simulink model "UWSim_test"  (R2018b)
settings: Solver=VariableStepAuto  StartTime=0.0  StopTime=10.0  RelTol=1e-3
libraries: simulink x6, robotlib x4
settings Model: Creator=carter  LastModifiedBy=carter

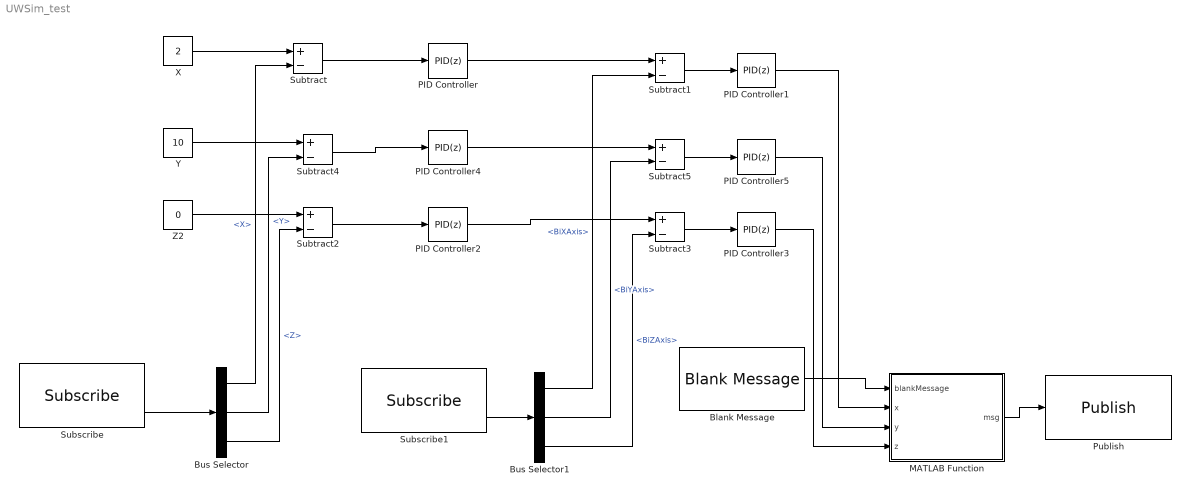
== system UWSim_test ==
  Blank Message : robotlib/Blank Message  messageClass=Message  entityType=std_msgs/Float64MultiArray  messageType=std_msgs/Float64MultiArray  SampleTime=1/50
      settings: SourceProductBaseCode=RO
  Bus Selector : BusSelector  OutputSignals=Position.X,Position.Y,Position.Z
  Bus Selector1 : BusSelector  OutputSignals=BiXAxis,BiYAxis,BiZAxis
  MATLAB Function : MATLAB Function  TreatAsAtomicUnit=on
  PID Controller{,1..5} (6 alike) : simulink/Continuous/PID Controller  Controller=PID  Form=Parallel  TimeDomain=Discrete-time  SampleTime=1/50  IntegratorMethod=Forward Euler  FilterMethod=Forward Euler  ControllerParametersSource=internal  P=0.5  I=0  D=0  UseFilter=on  N=100  TunerSelectOption=Transfer Function Based (PID Tuner App)  InitialConditionSource=internal  InitialConditionForIntegrator=0  InitialConditionForFilter=0  DifferentiatorICPrevScaledInput=0  ExternalReset=none  TrackingMode=off  Kt=1  LimitOutput=off  UpperSaturationLimit=inf  LowerSaturationLimit=-inf  LinearizeAsGain=on  AntiWindupMode=none  Kb=1  POutMin=[]  POutMax=[]  IOutMin=[]  IOutMax=[]  DOutMin=[]  DOutMax=[]  NOutMin=[]  NOutMax=[]  SumOutMin=[]  SumOutMax=[]  SaturationOutMin=[]  SaturationOutMax=[]  PParamMin=[]  PParamMax=[]  IParamMin=[]  IParamMax=[]  DParamMin=[]  DParamMax=[]  NParamMin=[]  NParamMax=[]  KbParamMin=[]  KbParamMax=[]  KtParamMin=[]  KtParamMax=[]  KbOutMin=[]  KbOutMax=[]  KtOutMin=[]  KtOutMax=[]  IntegratorOutMin=[]  IntegratorOutMax=[]  FilterOutMin=[]  FilterOutMax=[]  SumI1OutMin=[]  SumI1OutMax=[]  SumI2OutMin=[]  SumI2OutMax=[]  SumI3OutMin=[]  SumI3OutMax=[]  SumI4OutMin=[]  SumI4OutMax=[]  SumDOutMin=[]  SumDOutMax=[]  DifferentiatorOutMin=[]  DifferentiatorOutMax=[]  FilterDiffOutCoefMin=[]  FilterDiffOutCoefMax=[]  ReciprocalOutMin=[]  ReciprocalOutMax=[]  SumDenOutMin=[]  SumDenOutMax=[]  SumNumOutMin=[]  SumNumOutMax=[]  DivideOutMin=[]  DivideOutMax=[]  IntegratorContinuousStateAttributes=''  IntegratorStateMustResolveToSignalObject=off  IntegratorRTWStateStorageClass=Auto  FilterContinuousStateAttributes=''  FilterStateMustResolveToSignalObject=off  FilterRTWStateStorageClass=Auto  ParallelPVariant=InternalParameters  IdealPVariant=Disabled  IVariant=InternalParameters  DVariant=InternalParameters  IntegratorVariant=Discrete  SatVariant=Disabled  AWVariant=Passthrough  PCopyVariant=Disabled  TRVariant=Disabled  FdbkBlocksVariant=Forward  IdealPFdbkVariant=Disabled  SatFdbkVariant=Disabled  DerivativeFilterVariant=ForwardEulerFilter  NVariant=InternalParameters  NCopyVariant=Disabled  FilterICVariant=InternalICsFilter  IntegratorICVariant=InternalICs  ExternalResetVariant=Disabled  TRSumVariant=Passthrough  SumFdbkVariant=Disabled  SumVariant=Sum_PID
  Publish : robotlib/Publish  topicSource=Select from ROS network  topic=/g500/thrusters_input  messageType=std_msgs/Float64MultiArray  messageQueueLength=1
      settings: SourceProductBaseCode=RO
  Subscribe : robotlib/Subscribe  topicSource=Select from ROS network  topic=/g500/pose  messageType=geometry_msgs/Pose  sampleTime=1/50  messageQueueLength=1
      settings: SourceProductBaseCode=RO
  Subscribe1 : robotlib/Subscribe  topicSource=Select from ROS network  topic=/g500/dvl  messageType=underwater_sensor_msgs/DVL  sampleTime=1/50  messageQueueLength=1
      settings: SourceProductBaseCode=RO
  Subtract{,1..5} (6 alike) : Sum  Inputs=+-
  X : Constant  Value=2
  Y : Constant  Value=10
  "Z2 " : Constant  Value=0
  wires:
  Bus Selector/1 -> Subtract/2  "<X>"
  Subscribe/2 -> Bus Selector/1
  Bus Selector/2 -> Subtract4/2  "<Y>"
  X/1 -> Subtract/1
  Subtract/1 -> PID Controller/1
  Subscribe1/2 -> Bus Selector1/1
  Bus Selector1/1 -> Subtract1/2  "<BiXAxis>"
  PID Controller/1 -> Subtract1/1
  Subtract1/1 -> PID Controller1/1
  PID Controller1/1 -> MATLAB Function/2(x)
  Blank Message/1 -> MATLAB Function/1(blankMessage)
  MATLAB Function/1(msg) -> Publish/1
  Y/1 -> Subtract4/1
  "Z2 "/1 -> Subtract2/1
  Bus Selector/3 -> Subtract2/2  "<Z>"
  Subtract4/1 -> PID Controller4/1
  Subtract2/1 -> PID Controller2/1
  PID Controller4/1 -> Subtract5/1
  PID Controller2/1 -> Subtract3/1
  Bus Selector1/2 -> Subtract5/2  "<BiYAxis>"
  Bus Selector1/3 -> Subtract3/2  "<BiZAxis>"
  Subtract3/1 -> PID Controller3/1
  Subtract5/1 -> PID Controller5/1
  PID Controller5/1 -> MATLAB Function/3(y)
  PID Controller3/1 -> MATLAB Function/4(z)

== matlab function UWSim_test/MATLAB Function ==
  data: blankMessage input; msg output Bus: SL_Bus_UWSim_test_std_msgs_Float64MultiArray; x input; y input; z input
function msg = thrustersMap(blankMessage, x, y, z)
    % Assign the output message to be the same with input blank message
    msg = blankMessage;

    % Modify the nested message
    msg.Data(1) = -y;
    msg.Data(2) = -y;
    msg.Data(3) = -z;
    msg.Data(4) = -z;
    msg.Data(5) = -x;

    msg.Data_SL_Info.CurrentLength = uint32(5);
    disp(msg)
